simulink model "soal1ghesmateca"  (R2019b)
settings: Solver=VariableStepAuto  StartTime=0.0  StopTime=10  RelTol=1e-3
libraries: simulink x1
settings Model: Creator=user  LastModifiedBy=user

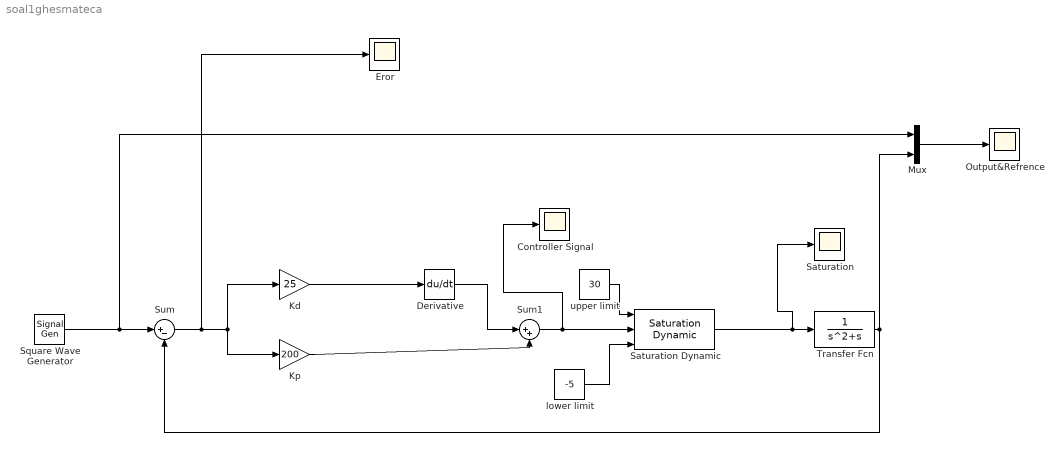
== system soal1ghesmateca ==
  "Controller Signal " : Scope
  Derivative : Derivative
  "Eror " : Scope
  "Kd " : Gain  Gain=25
  Kp : Gain  Gain=200
  Mux : Mux  Inputs=2
  Output&Refrence : Scope
  "Saturation " : Scope
  Saturation Dynamic : simulink/Discontinuities/Saturation Dynamic  OutMin=[]  OutMax=[]  OutDataTypeStr=Inherit: Same as second input  OutDataType=fixdt(1, 16)  OutScaling=2^-10  DoSatur=off
  "Square Wave Generator " : SignalGenerator  WaveForm=square  Amplitude=10  Frequency=2.5  Units=rad/sec
  Sum : Sum  Inputs=|+-
  Sum1 : Sum  Inputs=|++
  Transfer Fcn : TransferFcn  Denominator=[1 1 0]
  "lower limit " : Constant  Value=-5
  "upper limit " : Constant  Value=30
  wires:
  Derivative/1 -> Sum1/1
  Kp/1 -> Sum1/2
  "Kd "/1 -> Derivative/1
  "Square Wave Generator "/1 -> Mux/1, Sum/1
  Transfer Fcn/1 -> Sum/2, Mux/2
  Sum/1 -> "Eror "/1, Kp/1, "Kd "/1
  Saturation Dynamic/1 -> "Saturation "/1, Transfer Fcn/1
  "lower limit "/1 -> Saturation Dynamic/3
  "upper limit "/1 -> Saturation Dynamic/1
  Mux/1 -> Output&Refrence/1
  Sum1/1 -> "Controller Signal "/1, Saturation Dynamic/2
